simulink model "buck_pv_otm_MPPT2"  (R2024a)
settings: Solver=FixedStepAuto  StartTime=0  StopTime=0.8  FixedStep=(1/150000)/3  RelTol=1e-3
model workspace (MAT data in the model file):
  Var = 20
undefined symbols (not defined in the file or in its folder): kdE, kE, ki, ki_0, kki, kkp, kp, kp_0, n_pontos
libraries: spsSeriesRLCBranchLib x3, spsCurrentMeasurementLib x2, spsDiodeLib x2, spsMeanLib x2, simulink x1, spsDCVoltageSourceLib x1, spsGroundLib x1, spsMosfetLib x1, spsPVArrayLib x1, spsPWMGeneratorDCDCLib x1, spsVoltageMeasurementLib x1, spspowerguiLib x1
settings Model: Creator=mario  LastModifiedBy=UTFPR
settings SolverCC: MaxConsecutiveMinStep=10  ZeroCrossAlgorithm=Adaptive  SolverResetMethod=Robust
settings DebuggingCC: IgnoredZcDiagnostic=none
settings ModelReferenceCC: EnableRefExpFcnMdlSchedulingChecks=on
settings RTWCC: GPUComputeCapability=3.5

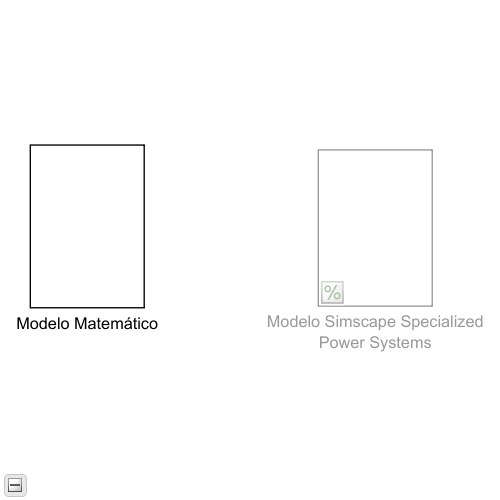
[thumbnail: Simulink's stored preview of the top-level diagram]
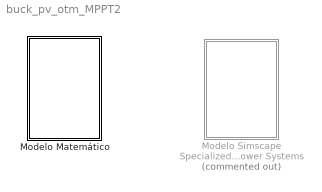
== system buck_pv_otm_MPPT2 ==
  Modelo Matemático : Subsystem
  Modelo Simscape Specialized Power Systems : Subsystem  Commented=on

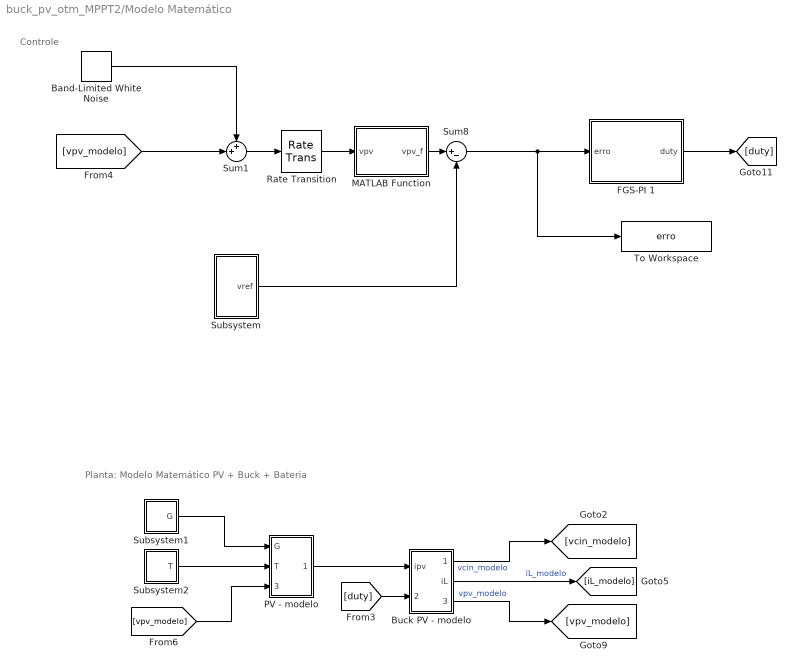
== system buck_pv_otm_MPPT2/Modelo Matemático ==
  note: Controle
  note: Planta: Modelo Matemático PV + Buck + Bateria
  Band-Limited White Noise : simulink/Sources/Band-Limited White Noise  Cov=[5e-7]  Ts=(1/150000)  seed=[23341]
  Buck PV - modelo : Subsystem
  FGS-PI 1 : Subsystem
  MATLAB Function : MATLAB Function  TreatAsAtomicUnit=on
  PV - modelo : Subsystem
  Rate Transition : RateTransition  OutPortSampleTime=1/150000
  Subsystem : Subsystem
  Subsystem1 : Subsystem
  Subsystem2 : Subsystem
  Sum1 : Sum  Inputs=++|
  Sum8 : Sum  Inputs=|+-
  To Workspace : ToWorkspace  VariableName=erro  SaveFormat=Timeseries  SampleTime=-1
  wires:
  [duty] -> Buck PV - modelo/2(duty)
  FGS-PI 1/1(duty) -> [duty]
  Buck PV - modelo/3(vpv) -> [vpv_modelo]  "vpv_modelo"
  Sum8/1 -> To Workspace/1, FGS-PI 1/1(erro)
  Buck PV - modelo/1(vcin) -> [vcin_modelo]  "vcin_modelo"
  Buck PV - modelo/2(iL) -> [iL_modelo]  "iL_modelo"
  [vpv_modelo] -> PV - modelo/3(Vpv)
  PV - modelo/1(Ipv) -> Buck PV - modelo/1(ipv)
  [vpv_modelo] -> Sum1/2
  Band-Limited White Noise/1 -> Sum1/1
  Sum1/1 -> Rate Transition/1
  MATLAB Function/1(vpv_f) -> Sum8/1
  Rate Transition/1 -> MATLAB Function/1(vpv)
  Subsystem/1(vref) -> Sum8/2
  Subsystem1/1(G) -> PV - modelo/1(G)
  Subsystem2/1(T) -> PV - modelo/2(T)

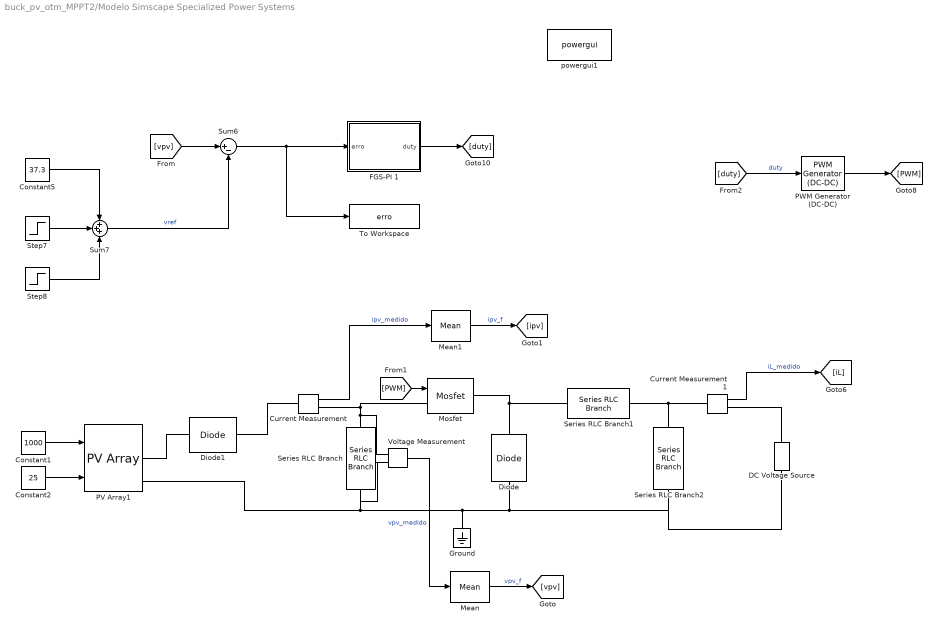
== system buck_pv_otm_MPPT2/Modelo Simscape Specialized Power Systems ==
  Constant1 : Constant  Value=1000
  Constant2 : Constant  Value=25
  Constant5 : Constant  Value=37.3
  Current Measurement : spsCurrentMeasurementLib/Current Measurement  PhasorSimulation=off  OutputType=Complex  PSBequivalent=0
  Current Measurement1 : spsCurrentMeasurementLib/Current Measurement  PhasorSimulation=off  OutputType=Complex  PSBequivalent=0
  DC Voltage Source : spsDCVoltageSourceLib/DC Voltage Source  Amplitude=12  Measurements=None
  Diode : spsDiodeLib/Diode  Ron=0.001  Lon=0  Vf=1  IC=0  UseSnubber=0  Rs=500  Cs=250e-9  Measurements=off
  Diode1 : spsDiodeLib/Diode  Ron=0.001  Lon=0  Vf=0.01  IC=0  UseSnubber=0  Rs=500  Cs=250e-9  Measurements=off
  FGS-PI 1 : Subsystem
  Ground : spsGroundLib/Ground  LConnTagsString=a
  Mean : spsMeanLib/Mean  Freq=150e2  Vinit=0  Ts=1e-7
  Mean1 : spsMeanLib/Mean  Freq=150e2  Vinit=0  Ts=1e-7
  Mosfet : spsMosfetLib/Mosfet  Ron=6.5e-3  Lon=0  Rd=0.01  Vfd=0  IC=0  Rs=1e5  Cs=inf  Measurements=off
  PV Array1 : spsPVArrayLib/PV Array  Npar=1  Nser=1  PlotType=array @ 1000 W/m2 & specified temperatures  S_vec="[ 1000  500  100 ]"  Temp_C_vec=[ 50 40 30 20 10 ]  ModuleName=User-defined  PlotWhenSelected=off  Pm=330.105  Ncell=72  Voc=46.1  Isc=9.29  Vm=37.3  Im=8.85  beta_Voc_pc=-0.32  alpha_Isc_pc=0.05  beta_Voc=-0.14752  alpha_Isc=0.004645  IL=9.3231  I0=7.1464e-11  nI=0.97384  Rsh=1329.6875  Rs=0.38666  RobustModel=off  RobustCellTemperature=313.3991  BAL=off  Tc=1e-7  Tfilter=6e-6
  PWM Generator (DC-DC) : spsPWMGeneratorDCDCLib/PWM Generator (DC-DC)  Fsw=150000  Ts=1e-7
  Series RLC Branch : spsSeriesRLCBranchLib/Series RLC Branch  LConnTagsString=__new0  RConnTagsString=__new0  BranchType=RC  Resistance=6.519e-3  Inductance=1e-3  SetiL0=off  InitialCurrent=0  Capacitance=2.7e-3  Setx0=on  InitialVoltage=0  Measurements=None
  Series RLC Branch1 : spsSeriesRLCBranchLib/Series RLC Branch  LConnTagsString=__new0  RConnTagsString=__new0  BranchType=RL  Resistance=3e-3  Inductance=22.109e-6  SetiL0=on  InitialCurrent=0  Capacitance=1e-6  Setx0=off  InitialVoltage=0  Measurements=None
  Series RLC Branch2 : spsSeriesRLCBranchLib/Series RLC Branch  LConnTagsString=__new0  RConnTagsString=__new0  BranchType=RC  Resistance=35.2e-3  Inductance=1e-3  SetiL0=off  InitialCurrent=0  Capacitance=500e-6  Setx0=on  InitialVoltage=0  Measurements=None
  Step7 : Step  Time=0.1  After=3  SampleTime=0
  Step8 : Step  Time=0.2  After=-3  SampleTime=0
  Sum6 : Sum  Inputs=|+-
  Sum7 : Sum  Inputs=+++
  To Workspace : ToWorkspace  VariableName=erro  SaveFormat=Timeseries  SampleTime=-1
  Voltage Measurement : spsVoltageMeasurementLib/Voltage Measurement  PhasorSimulation=off  OutputType=Complex  PSBequivalent=0
  powergui1 : spspowerguiLib/powergui  Priority=1  SimulationMode=Discrete  SampleTime=1e-7  frequency=60  Iterations=50  frequencyindice=0  Pbase=100e6  ErrMax=1e-4  UnitsV=kV  UnitsW=MW  buscounter=0  FunctionMessages=off  echomessages=off  EnableUseOfTLC=off  CurrentSourceSwitches=off  DisableSnubberDevices=on  DisableRonSwitches=off  DisableVfSwitches=off  DisplayEquations=off  AutomaticDiscreteSolvers=off  SolverType=Tustin/Backward Euler (TBE)  Interpol=off  ExternalGateDelay=off  methode=off  Ts=100  x0status=blocks  SPID=on  SwTol=0  HookPort=off  NonlinearTolerance=1e-4  nMaxIteration=100  ContinueOnMaxIteration=on  RestoreLinks=warning  ResistiveCurrentMeasurement=off  Frange=[0:2:500]  Ylog=off  Xlog=on  ShowGrid=off  save=off  variable=ZData  structure=0  ZoomFFT=off  StartTime=0.0  cycles=1  DisplayStyle=1  fundamental=60  FreqAxis=off  MaxFrequency=1000  frequencyindicesteady=1  RmsSteady=1  display=off
  wires:
  Current Measurement1/1 -> [iL]  "iL_medido"
  [duty] -> PWM Generator (DC-DC)/1  "duty"
  PWM Generator (DC-DC)/1 -> [PWM]
  [PWM] -> Mosfet/1
  [vpv] -> Sum6/1
  Step8/1 -> Sum7/3
  Step7/1 -> Sum7/2
  Constant5/1 -> Sum7/1
  Current Measurement/1 -> Mean1/1  "ipv_medido"
  Mean/1 -> [vpv]  "vpv_f"
  Voltage Measurement/1 -> Mean/1  "vpv_medido"
  FGS-PI 1/1(duty) -> [duty]
  Mean1/1 -> [ipv]  "ipv_f"
  Sum6/1 -> FGS-PI 1/1(erro), To Workspace/1
  Constant1/1 -> PV Array1/1
  Constant2/1 -> PV Array1/2
  Sum7/1 -> Sum6/2  "vref"
  connections:
  Series RLC Branch1/RConn1 -- Series RLC Branch2/LConn1 -- Current Measurement1/LConn1
  Voltage Measurement/LConn1 -- Mosfet/LConn1 -- Current Measurement/RConn1 -- Series RLC Branch/LConn1
  Ground/LConn1 -- PV Array1/RConn2 -- Series RLC Branch/RConn1 -- Voltage Measurement/LConn2 -- Series RLC Branch2/RConn1 -- DC Voltage Source/LConn1 -- Diode/LConn1
  Mosfet/RConn1 -- Series RLC Branch1/LConn1 -- Diode/RConn1
  Current Measurement1/RConn1 -- DC Voltage Source/RConn1
  Diode1/LConn1 -- PV Array1/RConn1
  Diode1/RConn1 -- Current Measurement/LConn1

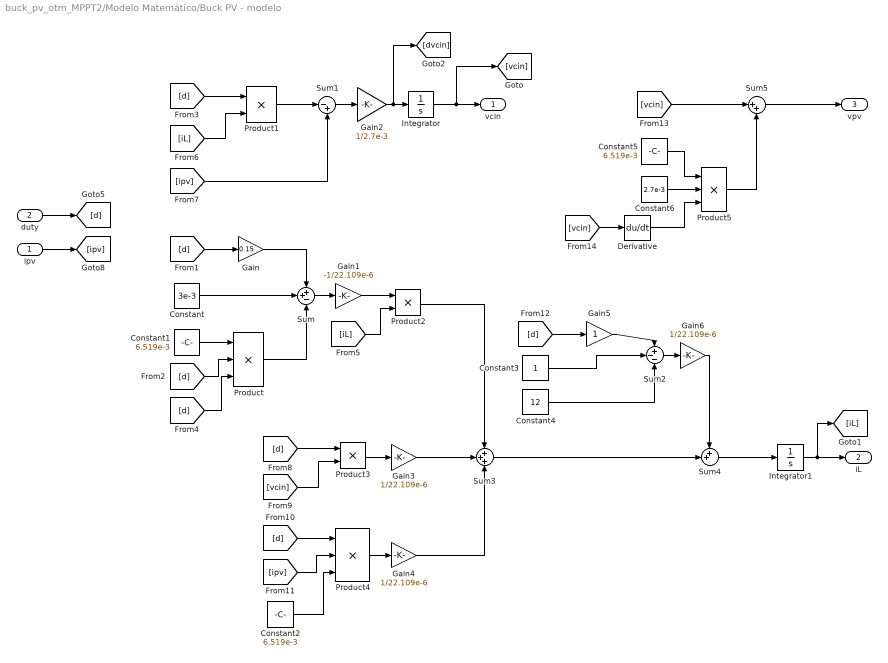
== system buck_pv_otm_MPPT2/Modelo Matemático/Buck PV - modelo ==
  ipv : Inport
  duty : Inport  Port=2
  Constant : Constant  Value=3e-3
  Constant1 : Constant  Value=6.519e-3
  Constant2 : Constant  Value=6.519e-3
  Constant3 : Constant
  Constant4 : Constant  Value=12
  Constant5 : Constant  Value=6.519e-3
  Constant6 : Constant  Value=2.7e-3
  Derivative : Derivative
  Gain : Gain  Gain=0.15
  Gain1 : Gain  Gain=-1/22.109e-6
  Gain2 : Gain  Gain=1/2.7e-3
  Gain3 : Gain  Gain=1/22.109e-6
  Gain4 : Gain  Gain=1/22.109e-6
  Gain5 : Gain
  Gain6 : Gain  Gain=1/22.109e-6
  Integrator : Integrator
  Integrator1 : Integrator
  Product : Product  Inputs=3
  Product1 : Product
  Product2 : Product
  Product3 : Product
  Product4 : Product  Inputs=3
  Product5 : Product  Inputs=3
  Sum : Sum  Inputs=++-
  Sum1 : Sum  Inputs=|-+
  Sum2 : Sum  Inputs=+--
  Sum3 : Sum  Inputs=+++
  Sum4 : Sum  Inputs=++|
  Sum5 : Sum  Inputs=|++
  vcin : Outport
  iL : Outport  Port=2
  vpv : Outport  Port=3
  wires:
  ipv/1 -> [ipv]
  [d] -> Product1/1
  Constant3/1 -> Sum2/2
  Product4/1 -> Gain4/1
  Constant2/1 -> Product4/3
  Sum1/1 -> Gain2/1
  [ipv] -> Product4/2
  Product3/1 -> Gain3/1
  [d] -> Product4/1
  Derivative/1 -> Product5/3
  Gain5/1 -> Sum2/1
  Sum5/1 -> vpv/1
  Constant1/1 -> Product/1
  [d] -> Product/3
  [d] -> Product/2
  Product/1 -> Sum/3
  [vcin] -> Sum5/1
  Constant5/1 -> Product5/1
  Product2/1 -> Sum3/1
  [d] -> Gain5/1
  Gain1/1 -> Product2/1
  Sum4/1 -> Integrator1/1
  Gain/1 -> Sum/1
  Product5/1 -> Sum5/2
  Sum3/1 -> Sum4/2
  [vcin] -> Derivative/1
  Integrator1/1 -> [iL], iL/1
  Constant4/1 -> Sum2/3
  Gain6/1 -> Sum4/1
  duty/1 -> [d]
  [vcin] -> Product3/2
  [d] -> Product3/1
  Sum2/1 -> Gain6/1
  Sum/1 -> Gain1/1
  [iL] -> Product2/2
  Constant/1 -> Sum/2
  Gain4/1 -> Sum3/3
  [d] -> Gain/1
  [iL] -> Product1/2
  Constant6/1 -> Product5/2
  Product1/1 -> Sum1/1
  Gain3/1 -> Sum3/2
  [ipv] -> Sum1/2
  Gain2/1 -> [dvcin], Integrator/1
  Integrator/1 -> [vcin], vcin/1

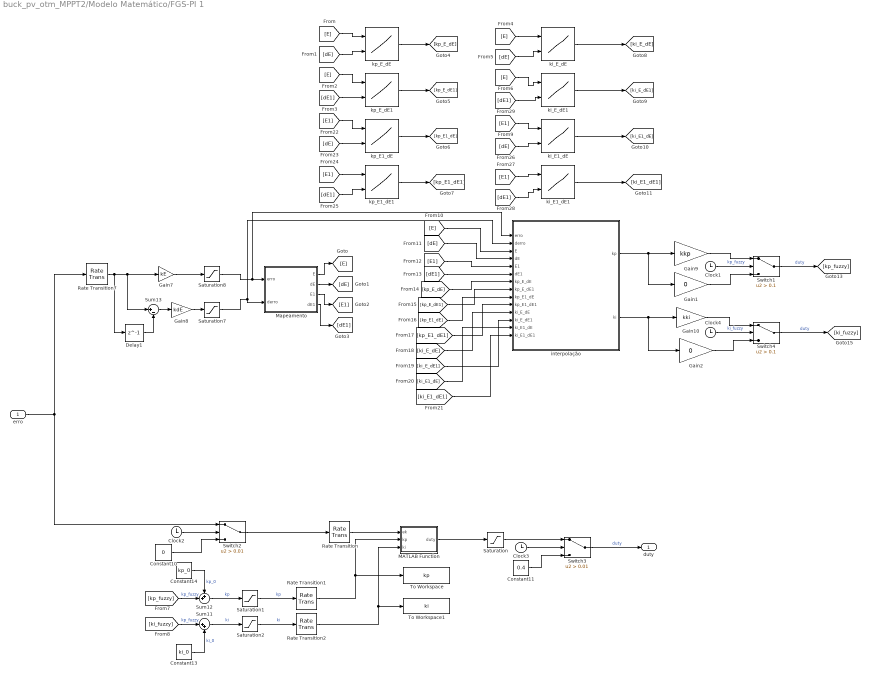
== system buck_pv_otm_MPPT2/Modelo Matemático/FGS-PI 1 ==
  erro : Inport
  Clock{1..4} (4 alike) : Clock
  Constant10 : Constant  Value=0
  Constant11 : Constant  Value=0.4
  Constant13 : Constant  Value=ki_0
  Constant14 : Constant  Value=kp_0
  Delay1 : Delay  DelayLength=1
  Gain1 : Gain  Gain=0
  Gain10 : Gain  Gain=kki
  Gain2 : Gain  Gain=0
  Gain7 : Gain  Gain=kE
  Gain8 : Gain  Gain=kdE
  Gain9 : Gain  Gain=kkp
  MATLAB Function : MATLAB Function  TreatAsAtomicUnit=on
  Mapeamento : MATLAB Function  TreatAsAtomicUnit=on
  Rate Transition : RateTransition  OutPortSampleTime=(1/150000)
  Rate Transition1 : RateTransition  OutPortSampleTime=(1/150000)
  Rate Transition2 : RateTransition  OutPortSampleTime=(1/150000)
  Rate Transition7 : RateTransition  OutPortSampleTime=(1/150000)*3
  Saturation : Saturate  UpperLimit=1  LowerLimit=0
  Saturation1 : Saturate  UpperLimit=10  LowerLimit=0
  Saturation2 : Saturate  UpperLimit=10  LowerLimit=0
  Saturation7 : Saturate  UpperLimit=1  LowerLimit=-1
  Saturation8 : Saturate  UpperLimit=1  LowerLimit=-1
  Sum11 : Sum  Inputs=|++
  Sum12 : Sum  Inputs=++|
  Sum13 : Sum  Inputs=|+-
  Switch1 : Switch  Criteria=u2 > Threshold  Threshold=0.1  SaturateOnIntegerOverflow=off  InputSameDT=off
  Switch2 : Switch  Criteria=u2 > Threshold  Threshold=0.01  SaturateOnIntegerOverflow=off  InputSameDT=off
  Switch3 : Switch  Criteria=u2 > Threshold  Threshold=0.01  SaturateOnIntegerOverflow=off  InputSameDT=off
  Switch4 : Switch  Criteria=u2 > Threshold  Threshold=0.1  SaturateOnIntegerOverflow=off  InputSameDT=off
  To Workspace : ToWorkspace  VariableName=kp  SaveFormat=Timeseries  SampleTime=-1
  To Workspace1 : ToWorkspace  VariableName=ki  SaveFormat=Timeseries  SampleTime=-1
  interpolação : MATLAB Function  TreatAsAtomicUnit=on
  ki_E1_dE : Lookup_n-D  LookupTableObject=''  BreakpointsForDimension1=[1:n_pontos+1]  BreakpointsForDimension2=[1:n_pontos+1]  BreakpointsForDimension1FirstPoint=10  BreakpointsForDimension2FirstPoint=10  BreakpointsForDimension1Spacing=12  BreakpointsForDimension2Spacing=12  IndexSearchMethod=Evenly spaced points  Table=ki  InterpMethod=Flat  DiagnosticForOutOfRangeInput=Error  InternalRulePriority=Speed  RndMeth=Simplest
      settings: InputPortMap=u0,u1
  ki_E1_dE1 : Lookup_n-D  LookupTableObject=''  BreakpointsForDimension1=[1:n_pontos+1]  BreakpointsForDimension2=[1:n_pontos+1]  BreakpointsForDimension1FirstPoint=10  BreakpointsForDimension2FirstPoint=10  BreakpointsForDimension1Spacing=12  BreakpointsForDimension2Spacing=12  IndexSearchMethod=Evenly spaced points  Table=ki  InterpMethod=Flat  DiagnosticForOutOfRangeInput=Error  InternalRulePriority=Speed  RndMeth=Simplest
      settings: InputPortMap=u0,u1
  ki_E_dE : Lookup_n-D  LookupTableObject=''  BreakpointsForDimension1=[1:n_pontos+1]  BreakpointsForDimension2=[1:n_pontos+1]  BreakpointsForDimension1FirstPoint=10  BreakpointsForDimension2FirstPoint=10  BreakpointsForDimension1Spacing=12  BreakpointsForDimension2Spacing=12  IndexSearchMethod=Evenly spaced points  Table=ki  InterpMethod=Flat  DiagnosticForOutOfRangeInput=Error  InternalRulePriority=Speed  RndMeth=Simplest
      settings: InputPortMap=u0,u1
  ki_E_dE1 : Lookup_n-D  LookupTableObject=''  BreakpointsForDimension1=[1:n_pontos+1]  BreakpointsForDimension2=[1:n_pontos+1]  BreakpointsForDimension1FirstPoint=10  BreakpointsForDimension2FirstPoint=10  BreakpointsForDimension1Spacing=12  BreakpointsForDimension2Spacing=12  IndexSearchMethod=Evenly spaced points  Table=ki  InterpMethod=Flat  DiagnosticForOutOfRangeInput=Error  InternalRulePriority=Speed  RndMeth=Simplest
      settings: InputPortMap=u0,u1
  kp_E1_dE : Lookup_n-D  LookupTableObject=''  BreakpointsForDimension1=[1:n_pontos+1]  BreakpointsForDimension2=[1:n_pontos+1]  BreakpointsForDimension1FirstPoint=10  BreakpointsForDimension2FirstPoint=10  BreakpointsForDimension1Spacing=12  BreakpointsForDimension2Spacing=12  IndexSearchMethod=Evenly spaced points  Table=kp  InterpMethod=Flat  DiagnosticForOutOfRangeInput=Error  InternalRulePriority=Speed  RndMeth=Simplest
      settings: InputPortMap=u0,u1
  kp_E1_dE1 : Lookup_n-D  LookupTableObject=''  BreakpointsForDimension1=[1:n_pontos+1]  BreakpointsForDimension2=[1:n_pontos+1]  BreakpointsForDimension1FirstPoint=10  BreakpointsForDimension2FirstPoint=10  BreakpointsForDimension1Spacing=12  BreakpointsForDimension2Spacing=12  IndexSearchMethod=Evenly spaced points  Table=kp  InterpMethod=Flat  DiagnosticForOutOfRangeInput=Error  InternalRulePriority=Speed  RndMeth=Simplest
      settings: InputPortMap=u0,u1
  kp_E_dE : Lookup_n-D  LookupTableObject=''  BreakpointsForDimension1=[1:n_pontos+1]  BreakpointsForDimension2=[1:n_pontos+1]  BreakpointsForDimension1FirstPoint=10  BreakpointsForDimension2FirstPoint=10  BreakpointsForDimension1Spacing=12  BreakpointsForDimension2Spacing=12  IndexSearchMethod=Evenly spaced points  Table=kp  InterpMethod=Flat  DiagnosticForOutOfRangeInput=Error  InternalRulePriority=Speed  RndMeth=Simplest
      settings: InputPortMap=u0,u1
  kp_E_dE1 : Lookup_n-D  LookupTableObject=''  BreakpointsForDimension1=[1:n_pontos+1]  BreakpointsForDimension2=[1:n_pontos+1]  BreakpointsForDimension1FirstPoint=10  BreakpointsForDimension2FirstPoint=10  BreakpointsForDimension1Spacing=12  BreakpointsForDimension2Spacing=12  IndexSearchMethod=Evenly spaced points  Table=kp  InterpMethod=Flat  DiagnosticForOutOfRangeInput=Error  InternalRulePriority=Speed  RndMeth=Simplest
      settings: InputPortMap=u0,u1
  duty : Outport
  wires:
  Saturation7/1 -> interpolação/2(derro), Mapeamento/2(derro)
  Saturation8/1 -> interpolação/1(erro), Mapeamento/1(erro)
  Sum13/1 -> Gain8/1
  Gain7/1 -> Saturation8/1
  Gain8/1 -> Saturation7/1
  Delay1/1 -> Sum13/2
  Constant13/1 -> Sum11/2  "ki_0"
  Rate Transition7/1 -> Delay1/1, Sum13/1, Gain7/1
  Rate Transition/1 -> MATLAB Function/1(ek)
  Sum12/1 -> Saturation1/1  "kp"
  Sum11/1 -> Saturation2/1  "ki"
  MATLAB Function/1(duty) -> Saturation/1
  Mapeamento/1(E) -> [E]
  Mapeamento/2(dE) -> [dE]
  Mapeamento/3(E1) -> [E1]
  Mapeamento/4(dE1) -> [dE1]
  interpolação/1(kp) -> Gain1/1, Gain9/1
  kp_E_dE/1 -> [kp_E_dE]
  kp_E_dE1/1 -> [kp_E_dE1]
  kp_E1_dE/1 -> [kp_E1_dE]
  kp_E1_dE1/1 -> [kp_E1_dE1]
  ki_E_dE/1 -> [ki_E_dE]
  ki_E_dE1/1 -> [ki_E_dE1]
  ki_E1_dE/1 -> [ki_E1_dE]
  ki_E1_dE1/1 -> [ki_E1_dE1]
  [E] -> interpolação/3(E)
  [dE] -> interpolação/4(dE)
  [E1] -> interpolação/5(E1)
  [dE1] -> interpolação/6(dE1)
  [kp_E_dE] -> interpolação/7(kp_E_dE)
  [kp_E_dE1] -> interpolação/8(kp_E_dE1)
  [kp_E1_dE] -> interpolação/9(kp_E1_dE)
  [kp_E1_dE1] -> interpolação/10(kp_E1_dE1)
  [ki_E_dE] -> interpolação/11(ki_E_dE)
  [ki_E_dE1] -> interpolação/12(ki_E_dE1)
  [ki_E1_dE] -> interpolação/13(ki_E1_dE)
  [ki_E1_dE1] -> interpolação/14(ki_E1_dE1)
  Constant14/1 -> Sum12/1  "kp_0"
  [kp_fuzzy] -> Sum12/2  "kp_fuzzy"
  [ki_fuzzy] -> Sum11/1  "kp_fuzzy"
  Constant10/1 -> Switch2/3
  erro/1 -> Switch2/1, Rate Transition7/1
  Clock2/1 -> Switch2/2
  Switch2/1 -> Rate Transition/1
  Saturation/1 -> Switch3/1
  Constant11/1 -> Switch3/3
  Clock3/1 -> Switch3/2
  Switch3/1 -> duty/1  "duty"
  Saturation1/1 -> Rate Transition1/1  "kp"
  Saturation2/1 -> Rate Transition2/1  "ki"
  Clock1/1 -> Switch1/2
  Gain9/1 -> Switch1/1  "kp_fuzzy"
  Switch1/1 -> [kp_fuzzy]  "duty"
  Gain1/1 -> Switch1/3
  Clock4/1 -> Switch4/2
  Switch4/1 -> [ki_fuzzy]  "duty"
  Gain10/1 -> Switch4/1  "ki_fuzzy"
  Gain2/1 -> Switch4/3
  interpolação/2(ki) -> Gain2/1, Gain10/1
  Rate Transition1/1 -> To Workspace/1, MATLAB Function/2(kp)
  Rate Transition2/1 -> To Workspace1/1, MATLAB Function/3(ki)
  [E] -> kp_E_dE/1
  [dE] -> kp_E_dE/2
  [E] -> kp_E_dE1/1
  [dE1] -> kp_E_dE1/2
  [E1] -> kp_E1_dE/1
  [dE] -> kp_E1_dE/2
  [E1] -> kp_E1_dE1/1
  [dE1] -> kp_E1_dE1/2
  [E] -> ki_E_dE/1
  [dE] -> ki_E_dE/2
  [E1] -> ki_E1_dE1/1
  [E1] -> ki_E1_dE/1
  [dE1] -> ki_E1_dE1/2
  [dE] -> ki_E1_dE/2
  [dE1] -> ki_E_dE1/2
  [E] -> ki_E_dE1/1

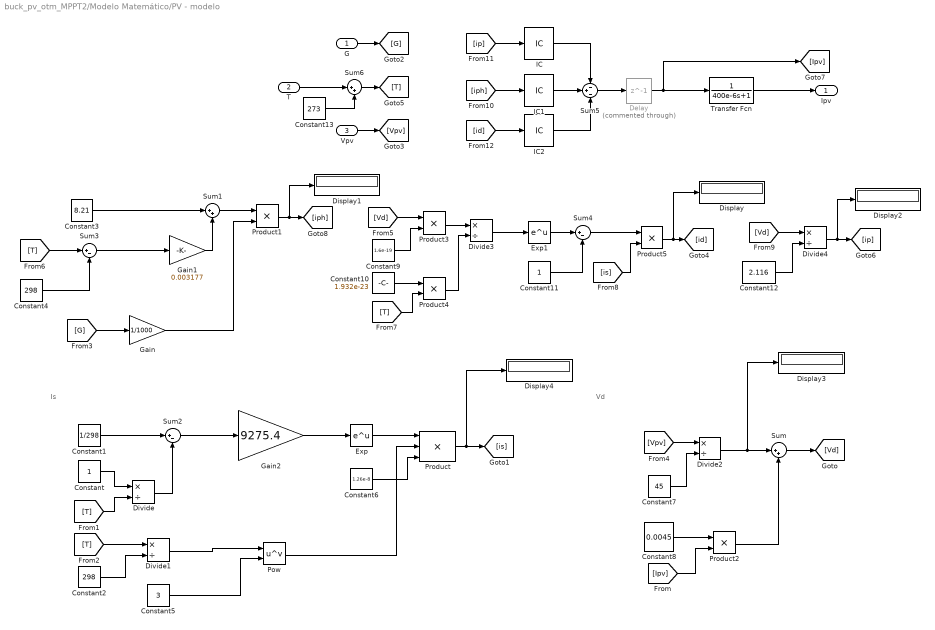
== system buck_pv_otm_MPPT2/Modelo Matemático/PV - modelo ==
  note: Is
  note: Vd
  G : Inport
  T : Inport  Port=2
  Vpv : Inport  Port=3
  Constant : Constant
  Constant1 : Constant  Value=1/298
  Constant10 : Constant  Value=1.932e-23
  Constant11 : Constant
  Constant12 : Constant  Value=2.116
  Constant13 : Constant  Value=273
  Constant2 : Constant  Value=298
  Constant3 : Constant  Value=8.21
  Constant4 : Constant  Value=298
  Constant5 : Constant  Value=3
  Constant6 : Constant  Value=1.26e-8
  Constant7 : Constant  Value=45
  Constant8 : Constant  Value=0.0045
  Constant9 : Constant  Value=1.6e-19
  Delay : Delay  Commented=through  DelayLength=1
  Display{,1..4} (5 alike) : Display
  Divide{,1..4} (5 alike) : Product  Inputs=*/
  Exp : Math
  Exp1 : Math
  Gain : Gain  Gain=1/1000
  Gain1 : Gain  Gain=0.003177
  Gain2 : Gain  Gain=9275.4
  IC : InitialCondition  Value=0
  IC1 : InitialCondition  Value=0
  IC2 : InitialCondition  Value=0
  Pow : Math  Operator=pow  SignedPower=on  RndMeth=Zero
  Product : Product  Inputs=3
  Product{1..5} (5 alike) : Product
  Sum : Sum  Inputs=|++
  Sum1 : Sum  Inputs=|++
  Sum2 : Sum  Inputs=|+-
  Sum3 : Sum  Inputs=|+-
  Sum4 : Sum  Inputs=|+-
  Sum5 : Sum  Inputs=-+-
  Sum6 : Sum  Inputs=|++
  Transfer Fcn : TransferFcn  Denominator=[400e-6 1]
  Ipv : Outport
  wires:
  [Ipv] -> Product2/2
  Constant7/1 -> Divide2/2
  Divide1/1 -> Pow/1
  Sum1/1 -> Product1/1
  [G] -> Gain/1
  Gain1/1 -> Sum1/2
  Sum3/1 -> Gain1/1
  [ip] -> IC/1
  Constant2/1 -> Divide1/2
  [T] -> Sum3/1
  T/1 -> Sum6/1
  Constant1/1 -> Sum2/1
  Constant13/1 -> Sum6/2
  Product1/1 -> Display1/1, [iph]
  Sum6/1 -> [T]
  G/1 -> [G]
  [Vd] -> Divide4/1
  IC/1 -> Sum5/1
  IC1/1 -> Sum5/2
  Product4/1 -> Divide3/2
  Product5/1 -> Display/1, [id]
  Constant/1 -> Divide/1
  Divide4/1 -> Display2/1, [ip]
  Delay/1 -> [Ipv], Transfer Fcn/1
  Divide3/1 -> Exp1/1
  Sum5/1 -> Delay/1
  Exp/1 -> Product/1
  [T] -> Divide1/1
  Gain2/1 -> Exp/1
  [Vpv] -> Divide2/1
  Constant10/1 -> Product4/1
  Constant6/1 -> Product/3
  Sum2/1 -> Gain2/1
  Pow/1 -> Product/2
  Sum4/1 -> Product5/1
  Constant11/1 -> Sum4/2
  [id] -> IC2/1
  Product/1 -> Display4/1, [is]
  Constant3/1 -> Sum1/1
  Constant12/1 -> Divide4/2
  Constant5/1 -> Pow/2
  Divide2/1 -> Display3/1, Sum/1
  [is] -> Product5/2
  Sum/1 -> [Vd]
  Exp1/1 -> Sum4/1
  IC2/1 -> Sum5/3
  Divide/1 -> Sum2/2
  Vpv/1 -> [Vpv]
  [T] -> Product4/2
  Gain/1 -> Product1/2
  Product3/1 -> Divide3/1
  [iph] -> IC1/1
  Constant9/1 -> Product3/2
  Constant4/1 -> Sum3/2
  [T] -> Divide/2
  Constant8/1 -> Product2/1
  [Vd] -> Product3/1
  Product2/1 -> Sum/2
  Transfer Fcn/1 -> Ipv/1

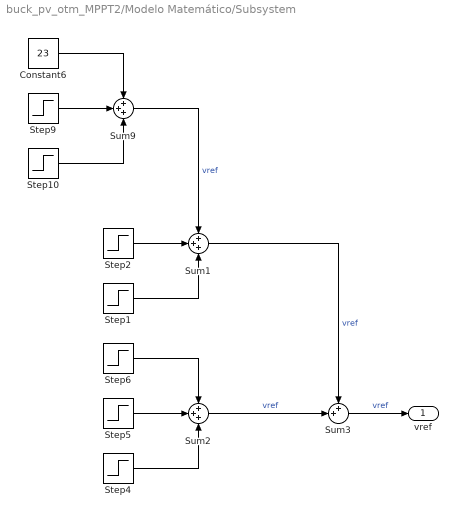
== system buck_pv_otm_MPPT2/Modelo Matemático/Subsystem ==
  Constant6 : Constant  Value=23
  Step1 : Step  Time=0.45  After=0.5  SampleTime=0
  Step10 : Step  Time=0.2  After=-3  SampleTime=0
  Step2 : Step  Time=0.35  After=2.7  SampleTime=0
  Step4 : Step  Time=0.75  After=-0.8  SampleTime=0
  Step5 : Step  Time=0.65  After=-0.3  SampleTime=0
  Step6 : Step  Time=0.55  After=-0.8  SampleTime=0
  Step9 : Step  Time=0.1  After=3  SampleTime=0
  Sum1 : Sum  Inputs=+++
  Sum2 : Sum  Inputs=+++
  Sum3 : Sum  Inputs=++|
  Sum9 : Sum  Inputs=+++
  vref : Outport
  wires:
  Step10/1 -> Sum9/3
  Constant6/1 -> Sum9/1
  Step9/1 -> Sum9/2
  Step1/1 -> Sum1/3
  Step2/1 -> Sum1/2
  Step6/1 -> Sum2/1
  Step4/1 -> Sum2/3
  Step5/1 -> Sum2/2
  Sum9/1 -> Sum1/1  "vref"
  Sum2/1 -> Sum3/2  "vref"
  Sum1/1 -> Sum3/1  "vref"
  Sum3/1 -> vref/1  "vref"

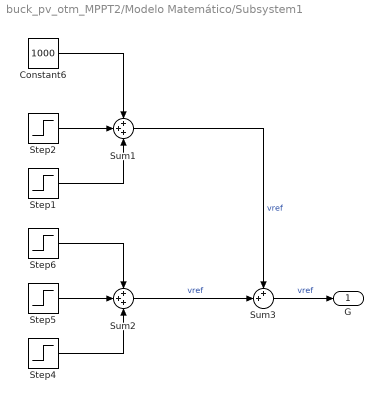
== system buck_pv_otm_MPPT2/Modelo Matemático/Subsystem1 ==
  Constant6 : Constant  Value=1000
  Step1 : Step  Time=0.4  After=(562-165)  SampleTime=0
  Step2 : Step  Time=0.3  After=(165-1000)  SampleTime=0
  Step4 : Step  Time=0.7  After=(186-570)  SampleTime=0
  Step5 : Step  Time=0.6  After=(570-767)  SampleTime=0
  Step6 : Step  Time=0.5  After=(767-562)  SampleTime=0
  Sum1 : Sum  Inputs=+++
  Sum2 : Sum  Inputs=+++
  Sum3 : Sum  Inputs=++|
  G : Outport
  wires:
  Sum3/1 -> G/1  "vref"
  Sum1/1 -> Sum3/1  "vref"
  Sum2/1 -> Sum3/2  "vref"
  Step5/1 -> Sum2/2
  Step4/1 -> Sum2/3
  Step6/1 -> Sum2/1
  Step2/1 -> Sum1/2
  Step1/1 -> Sum1/3
  Constant6/1 -> Sum1/1

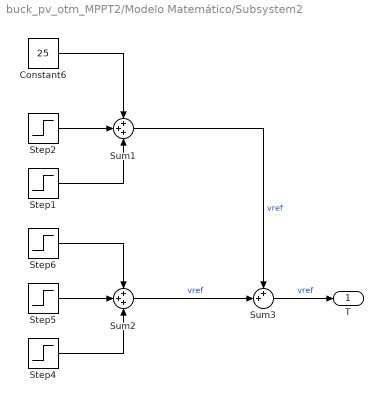
== system buck_pv_otm_MPPT2/Modelo Matemático/Subsystem2 ==
  Constant6 : Constant  Value=25
  Step1 : Step  Time=0.4  After=(27-12)  SampleTime=0
  Step2 : Step  Time=0.3  After=(12-25)  SampleTime=0
  Step4 : Step  Time=0.7  After=30-40  SampleTime=0
  Step5 : Step  Time=0.6  After=0  SampleTime=0
  Step6 : Step  Time=0.5  After=(40-27)  SampleTime=0
  Sum1 : Sum  Inputs=+++
  Sum2 : Sum  Inputs=+++
  Sum3 : Sum  Inputs=++|
  T : Outport
  wires:
  Constant6/1 -> Sum1/1
  Step1/1 -> Sum1/3
  Step2/1 -> Sum1/2
  Step6/1 -> Sum2/1
  Step4/1 -> Sum2/3
  Step5/1 -> Sum2/2
  Sum2/1 -> Sum3/2  "vref"
  Sum1/1 -> Sum3/1  "vref"
  Sum3/1 -> T/1  "vref"

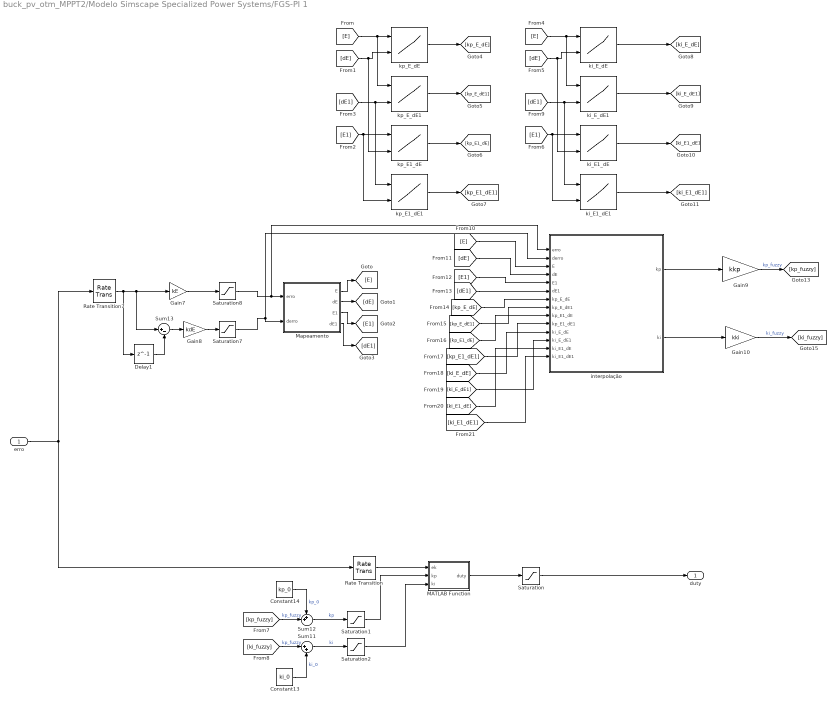
== system buck_pv_otm_MPPT2/Modelo Simscape Specialized Power Systems/FGS-PI 1 ==
  erro : Inport
  Constant13 : Constant  Value=ki_0
  Constant14 : Constant  Value=kp_0
  Delay1 : Delay  DelayLength=1
  Gain10 : Gain  Gain=kki
  Gain7 : Gain  Gain=kE
  Gain8 : Gain  Gain=kdE
  Gain9 : Gain  Gain=kkp
  MATLAB Function : MATLAB Function  TreatAsAtomicUnit=on
  Mapeamento : MATLAB Function  TreatAsAtomicUnit=on
  Rate Transition : RateTransition  OutPortSampleTime=1/100000
  Rate Transition7 : RateTransition  OutPortSampleTime=20e-6
  Saturation : Saturate  UpperLimit=1  LowerLimit=0
  Saturation1 : Saturate  UpperLimit=10  LowerLimit=0
  Saturation2 : Saturate  UpperLimit=10  LowerLimit=0
  Saturation7 : Saturate  UpperLimit=1  LowerLimit=-1
  Saturation8 : Saturate  UpperLimit=1  LowerLimit=-1
  Sum11 : Sum  Inputs=|++
  Sum12 : Sum  Inputs=++|
  Sum13 : Sum  Inputs=|+-
  interpolação : MATLAB Function  TreatAsAtomicUnit=on
  ki_E1_dE : Lookup_n-D  LookupTableObject=''  BreakpointsForDimension1=[1:n_pontos+1]  BreakpointsForDimension2=[1:n_pontos+1]  BreakpointsForDimension1FirstPoint=10  BreakpointsForDimension2FirstPoint=10  BreakpointsForDimension1Spacing=12  BreakpointsForDimension2Spacing=12  IndexSearchMethod=Evenly spaced points  Table=ki  InterpMethod=Flat  DiagnosticForOutOfRangeInput=Error  InternalRulePriority=Speed  RndMeth=Simplest
      settings: InputPortMap=u0,u1
  ki_E1_dE1 : Lookup_n-D  LookupTableObject=''  BreakpointsForDimension1=[1:n_pontos+1]  BreakpointsForDimension2=[1:n_pontos+1]  BreakpointsForDimension1FirstPoint=10  BreakpointsForDimension2FirstPoint=10  BreakpointsForDimension1Spacing=12  BreakpointsForDimension2Spacing=12  IndexSearchMethod=Evenly spaced points  Table=ki  InterpMethod=Flat  DiagnosticForOutOfRangeInput=Error  InternalRulePriority=Speed  RndMeth=Simplest
      settings: InputPortMap=u0,u1
  ki_E_dE : Lookup_n-D  LookupTableObject=''  BreakpointsForDimension1=[1:n_pontos+1]  BreakpointsForDimension2=[1:n_pontos+1]  BreakpointsForDimension1FirstPoint=10  BreakpointsForDimension2FirstPoint=10  BreakpointsForDimension1Spacing=12  BreakpointsForDimension2Spacing=12  IndexSearchMethod=Evenly spaced points  Table=ki  InterpMethod=Flat  DiagnosticForOutOfRangeInput=Error  InternalRulePriority=Speed  RndMeth=Simplest
      settings: InputPortMap=u0,u1
  ki_E_dE1 : Lookup_n-D  LookupTableObject=''  BreakpointsForDimension1=[1:n_pontos+1]  BreakpointsForDimension2=[1:n_pontos+1]  BreakpointsForDimension1FirstPoint=10  BreakpointsForDimension2FirstPoint=10  BreakpointsForDimension1Spacing=12  BreakpointsForDimension2Spacing=12  IndexSearchMethod=Evenly spaced points  Table=ki  InterpMethod=Flat  DiagnosticForOutOfRangeInput=Error  InternalRulePriority=Speed  RndMeth=Simplest
      settings: InputPortMap=u0,u1
  kp_E1_dE : Lookup_n-D  LookupTableObject=''  BreakpointsForDimension1=[1:n_pontos+1]  BreakpointsForDimension2=[1:n_pontos+1]  BreakpointsForDimension1FirstPoint=10  BreakpointsForDimension2FirstPoint=10  BreakpointsForDimension1Spacing=12  BreakpointsForDimension2Spacing=12  IndexSearchMethod=Evenly spaced points  Table=kp  InterpMethod=Flat  DiagnosticForOutOfRangeInput=Error  InternalRulePriority=Speed  RndMeth=Simplest
      settings: InputPortMap=u0,u1
  kp_E1_dE1 : Lookup_n-D  LookupTableObject=''  BreakpointsForDimension1=[1:n_pontos+1]  BreakpointsForDimension2=[1:n_pontos+1]  BreakpointsForDimension1FirstPoint=10  BreakpointsForDimension2FirstPoint=10  BreakpointsForDimension1Spacing=12  BreakpointsForDimension2Spacing=12  IndexSearchMethod=Evenly spaced points  Table=kp  InterpMethod=Flat  DiagnosticForOutOfRangeInput=Error  InternalRulePriority=Speed  RndMeth=Simplest
      settings: InputPortMap=u0,u1
  kp_E_dE : Lookup_n-D  LookupTableObject=''  BreakpointsForDimension1=[1:n_pontos+1]  BreakpointsForDimension2=[1:n_pontos+1]  BreakpointsForDimension1FirstPoint=10  BreakpointsForDimension2FirstPoint=10  BreakpointsForDimension1Spacing=12  BreakpointsForDimension2Spacing=12  IndexSearchMethod=Evenly spaced points  Table=kp  InterpMethod=Flat  DiagnosticForOutOfRangeInput=Error  InternalRulePriority=Speed  RndMeth=Simplest
      settings: InputPortMap=u0,u1
  kp_E_dE1 : Lookup_n-D  LookupTableObject=''  BreakpointsForDimension1=[1:n_pontos+1]  BreakpointsForDimension2=[1:n_pontos+1]  BreakpointsForDimension1FirstPoint=10  BreakpointsForDimension2FirstPoint=10  BreakpointsForDimension1Spacing=12  BreakpointsForDimension2Spacing=12  IndexSearchMethod=Evenly spaced points  Table=kp  InterpMethod=Flat  DiagnosticForOutOfRangeInput=Error  InternalRulePriority=Speed  RndMeth=Simplest
      settings: InputPortMap=u0,u1
  duty : Outport
  wires:
  Saturation7/1 -> interpolação/2(derro), Mapeamento/2(derro)
  Saturation8/1 -> interpolação/1(erro), Mapeamento/1(erro)
  Sum13/1 -> Gain8/1
  Gain7/1 -> Saturation8/1
  Gain9/1 -> [kp_fuzzy]  "kp_fuzzy"
  Gain8/1 -> Saturation7/1
  Delay1/1 -> Sum13/2
  Constant13/1 -> Sum11/2  "ki_0"
  Gain10/1 -> [ki_fuzzy]  "ki_fuzzy"
  Rate Transition7/1 -> Delay1/1, Sum13/1, Gain7/1
  Rate Transition/1 -> MATLAB Function/1(ek)
  Sum12/1 -> Saturation1/1  "kp"
  Sum11/1 -> Saturation2/1  "ki"
  MATLAB Function/1(duty) -> Saturation/1
  Mapeamento/1(E) -> [E]
  Mapeamento/2(dE) -> [dE]
  Mapeamento/3(E1) -> [E1]
  Mapeamento/4(dE1) -> [dE1]
  [E] -> kp_E_dE1/1, kp_E_dE/1
  [dE] -> kp_E1_dE/2, kp_E_dE/2
  [dE1] -> kp_E1_dE1/1, kp_E_dE1/2
  [E1] -> kp_E1_dE1/2, kp_E1_dE/1
  [E1] -> ki_E1_dE/1, ki_E1_dE1/2
  [dE1] -> ki_E_dE1/2, ki_E1_dE1/1
  [dE] -> ki_E_dE/2, ki_E1_dE/2
  [E] -> ki_E_dE/1, ki_E_dE1/1
  interpolação/1(kp) -> Gain9/1
  interpolação/2(ki) -> Gain10/1
  kp_E_dE/1 -> [kp_E_dE]
  kp_E_dE1/1 -> [kp_E_dE1]
  kp_E1_dE/1 -> [kp_E1_dE]
  kp_E1_dE1/1 -> [kp_E1_dE1]
  ki_E_dE/1 -> [ki_E_dE]
  ki_E_dE1/1 -> [ki_E_dE1]
  ki_E1_dE/1 -> [ki_E1_dE]
  ki_E1_dE1/1 -> [ki_E1_dE1]
  [E] -> interpolação/3(E)
  [dE] -> interpolação/4(dE)
  [E1] -> interpolação/5(E1)
  [dE1] -> interpolação/6(dE1)
  [kp_E_dE] -> interpolação/7(kp_E_dE)
  [kp_E_dE1] -> interpolação/8(kp_E_dE1)
  [kp_E1_dE] -> interpolação/9(kp_E1_dE)
  [kp_E1_dE1] -> interpolação/10(kp_E1_dE1)
  [ki_E_dE] -> interpolação/11(ki_E_dE)
  [ki_E_dE1] -> interpolação/12(ki_E_dE1)
  [ki_E1_dE] -> interpolação/13(ki_E1_dE)
  [ki_E1_dE1] -> interpolação/14(ki_E1_dE1)
  Constant14/1 -> Sum12/1  "kp_0"
  [kp_fuzzy] -> Sum12/2  "kp_fuzzy"
  [ki_fuzzy] -> Sum11/1  "kp_fuzzy"
  erro/1 -> Rate Transition/1, Rate Transition7/1
  Saturation1/1 -> MATLAB Function/2(kp)
  Saturation2/1 -> MATLAB Function/3(ki)
  Saturation/1 -> duty/1

== matlab function buck_pv_otm_MPPT2/Modelo Simscape Specialized Power Systems/FGS-PI 1/MATLAB Function ==
  settings: updateMethod=DISCRETE
  data: ek input; duty output; kp input; ki input
%% Discretização por Tustin do PI(z)
function duty = fcn(ek, kp, ki)

persistent uk_1 ek_1

if(isempty(uk_1)) uk_1=0; end
if(isempty(ek_1)) ek_1=0; end

Ts = (1/100e3);
A = kp + (ki*Ts/2);
B = kp - (ki*Ts/2);

u_PI = A*ek - B*ek_1 + uk_1;

ek_1 = ek;
uk_1 = u_PI;

duty = u_PI;

== matlab function buck_pv_otm_MPPT2/Modelo Simscape Specialized Power Systems/FGS-PI 1/Mapeamento ==
  data: erro input; E output; derro input; dE output; E1 output; dE1 output
function [E, dE, E1, dE1] = fcn(erro, derro)
   persistent ek_1;
   n_pontos = 20;

    if(isempty(ek_1)) ek_1=0; end

    E = (floor((n_pontos/2)*erro + (n_pontos/2)+1));
    dE = (floor((n_pontos/2)*derro + (n_pontos/2)+1));
    if(E+1 > n_pontos+1)
        E1 = E;
    else
        E1 = E+1;
    end

    if(dE+1 > n_pontos+1)
        dE1 = dE;
    else
        dE1 = dE+1;
    end

== matlab function buck_pv_otm_MPPT2/Modelo Simscape Specialized Power Systems/FGS-PI 1/interpolação ==
  data: erro input; kp output; derro input; ki output; E input; dE input; E1 input; dE1 input; kp_E_dE input; kp_E_dE1 input; kp_E1_dE input; kp_E1_dE1 input; ki_E_dE input; ki_E_dE1 input; ki_E1_dE input; ki_E1_dE1 input
function [kp, ki] = fcn(erro, derro, E, dE, E1, dE1, kp_E_dE, kp_E_dE1, kp_E1_dE, kp_E1_dE1, ki_E_dE, ki_E_dE1, ki_E1_dE, ki_E1_dE1)
    
    if (E == E1 || dE == dE1)
        kp = kp_E_dE;
        ki = ki_E_dE;
    else
        n = 20;
        erro_E = 2*E/n - (1+2/n);
        derro_dE = 2*dE/n - (1+2/n);
        erro_E1 = 2*E1/n - (1+2/n);
        derro_dE1 = 2*dE1/n - (1+2/n);
    
        kp_erro_dE = ((kp_E1_dE - kp_E_dE)/(erro_E1 - erro_E))*(erro-erro_E)+kp_E_dE;
        ki_erro_dE = ((ki_E1_dE - ki_E_dE)/(erro_E1 - erro_E))*(erro-erro_E)+ki_E_dE;
    
        kp_erro_dE1 = ((kp_E1_dE1 - kp_E_dE1)/(erro_E1-erro_E))*(erro-erro_E)+kp_E_dE1;
        ki_erro_dE1 = ((ki_E1_dE1 - ki_E_dE1)/(erro_E1-erro_E))*(erro-erro_E)+ki_E_dE1;
    
        kp = ((kp_erro_dE1 - kp_erro_dE)/(derro_dE1-derro_dE))*(derro-derro_dE) + kp_erro_dE;
        ki = ((ki_erro_dE1 - ki_erro_dE)/(derro_dE1-derro_dE))*(derro-derro_dE) + ki_erro_dE;
    end

== matlab function buck_pv_otm_MPPT2/Modelo Matemático/MATLAB Function ==
  data: vpv input; vpv_f output
function vpv_f = fcn(vpv)

% Valores p/ fc = 15 kHz
% b0 = 0.23905722;
% b1 = 0.23905722;
% a1 = -0.52188555;

% Valores p/ fc = 1.5 kHz
b0 = 0.030459028;
b1 = 0.030459028;
a1 = -0.93908194;

persistent vpv1 vpv_f1

if(isempty(vpv1)) vpv1=0; end
if(isempty(vpv_f1)) vpv_f1=0; end

vpv_f = (b0*vpv)+(b1*vpv1)-(a1*vpv_f1);
vpv1 = vpv;
vpv_f1 = vpv_f;

== matlab function buck_pv_otm_MPPT2/Modelo Matemático/FGS-PI 1/MATLAB Function ==
  settings: updateMethod=DISCRETE
  data: ek input; duty output; kp input; ki input
%% Discretização por Tustin do PI(z)
function duty = fcn(ek, kp, ki)

persistent uk_1 ek_1

if(isempty(uk_1)) uk_1=0; end
if(isempty(ek_1)) ek_1=0; end

Ts = (1/150e3);
A = kp + (ki*Ts/2);
B = kp - (ki*Ts/2);

u_PI = A*ek - B*ek_1 + uk_1;

ek_1 = ek;
uk_1 = u_PI;

duty = u_PI;

== matlab function buck_pv_otm_MPPT2/Modelo Matemático/FGS-PI 1/Mapeamento ==
  data: erro input; E output; derro input; dE output; E1 output; dE1 output
function [E, dE, E1, dE1] = fcn(erro, derro)
   persistent ek_1;
   n_pontos = 20;

    if(isempty(ek_1)) ek_1=0; end

    E = (floor((n_pontos/2)*erro + (n_pontos/2)+1));
    dE = (floor((n_pontos/2)*derro + (n_pontos/2)+1));
    if(E+1 > n_pontos+1)
        E1 = E;
    else
        E1 = E+1;
    end

    if(dE+1 > n_pontos+1)
        dE1 = dE;
    else
        dE1 = dE+1;
    end

== matlab function buck_pv_otm_MPPT2/Modelo Matemático/FGS-PI 1/interpolação ==
  data: erro input; kp output; derro input; ki output; E input; dE input; E1 input; dE1 input; kp_E_dE input; kp_E_dE1 input; kp_E1_dE input; kp_E1_dE1 input; ki_E_dE input; ki_E_dE1 input; ki_E1_dE input; ki_E1_dE1 input
function [kp, ki] = fcn(erro, derro, E, dE, E1, dE1, kp_E_dE, kp_E_dE1, kp_E1_dE, kp_E1_dE1, ki_E_dE, ki_E_dE1, ki_E1_dE, ki_E1_dE1)
    
    if (E == E1 || dE == dE1)
        kp = kp_E_dE;
        ki = ki_E_dE;
    else
        n = 20;
        erro_E = 2*E/n - (1+2/n);
        derro_dE = 2*dE/n - (1+2/n);
        erro_E1 = 2*E1/n - (1+2/n);
        derro_dE1 = 2*dE1/n - (1+2/n);
    
        kp_erro_dE = ((kp_E1_dE - kp_E_dE)/(erro_E1 - erro_E))*(erro-erro_E)+kp_E_dE;
        ki_erro_dE = ((ki_E1_dE - ki_E_dE)/(erro_E1 - erro_E))*(erro-erro_E)+ki_E_dE;
    
        kp_erro_dE1 = ((kp_E1_dE1 - kp_E_dE1)/(erro_E1-erro_E))*(erro-erro_E)+kp_E_dE1;
        ki_erro_dE1 = ((ki_E1_dE1 - ki_E_dE1)/(erro_E1-erro_E))*(erro-erro_E)+ki_E_dE1;
    
        kp = ((kp_erro_dE1 - kp_erro_dE)/(derro_dE1-derro_dE))*(derro-derro_dE) + kp_erro_dE;
        ki = ((ki_erro_dE1 - ki_erro_dE)/(derro_dE1-derro_dE))*(derro-derro_dE) + ki_erro_dE;
    end
